simulink model "Taller5"  (R2024a)
settings: Solver=ode4  StartTime=0.0  StopTime=0.050  FixedStep=1e-6  RelTol=1e-3
values from neighbouring files (symbols this model uses):
  den = [1, R/L, 1/(L * Cap)]    [Taller5_codigo.m]
  Kd3 = 0.0362210629547162    (= 0.0362210629547)    [Taller5_codigo.m]
  Ki2 = 500    [Taller5_codigo.m]
  Ki3 = 1762.80242907617    (= 1762.80242908)    [Taller5_codigo.m]
  Kp = 100    [Taller5_codigo.m]
  Kp2 = 10    [Taller5_codigo.m]
  Kp3 = 16.7573383387027    (= 16.7573383387)    [Taller5_codigo.m]
  num = 1/(L * Cap)    (= 45454.5454545)    [Taller5_codigo.m]
libraries: slpidlib x2
settings Model: Creator=UsuarioF  LastModifiedBy=UsuarioF

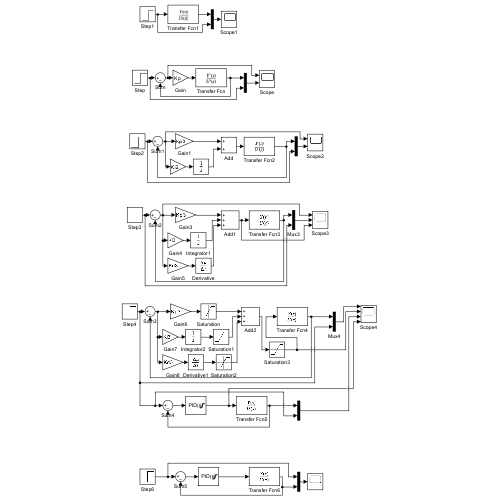
[thumbnail: Simulink's stored preview of the top-level diagram]
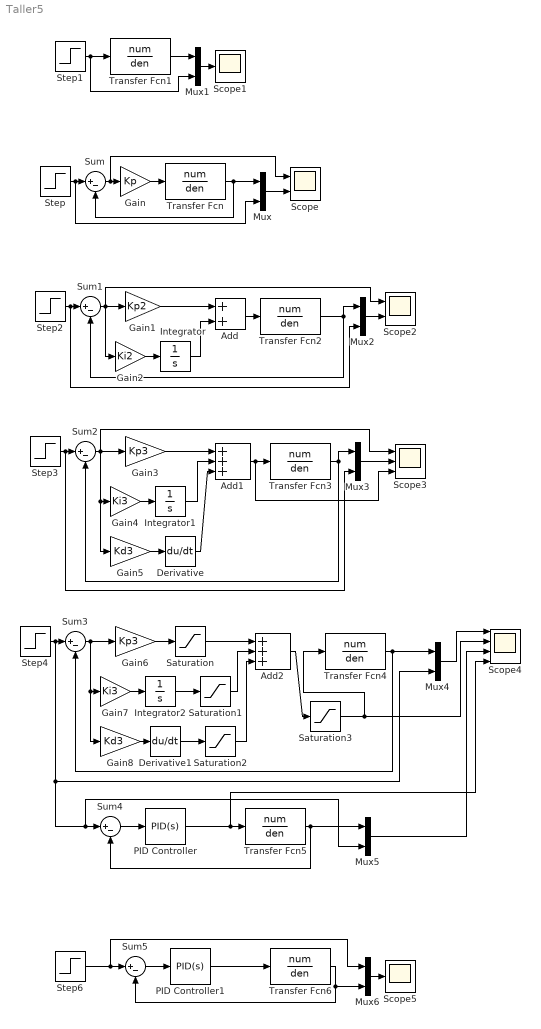
== system Taller5 ==
  Add : Sum
  Add1 : Sum  Inputs=+++
  Add2 : Sum  Inputs=+++
  Derivative : Derivative
  Derivative1 : Derivative
  Gain : Gain  Gain=Kp
  Gain1 : Gain  Gain=Kp2
  Gain2 : Gain  Gain=Ki2
  Gain3 : Gain  Gain=Kp3
  Gain4 : Gain  Gain=Ki3
  Gain5 : Gain  Gain=Kd3
  Gain6 : Gain  Gain=Kp3
  Gain7 : Gain  Gain=Ki3
  Gain8 : Gain  Gain=Kd3
  Integrator : Integrator
  Integrator1 : Integrator
  Integrator2 : Integrator
  Mux{,1..6} (7 alike) : Mux  Inputs=2
  PID Controller : slpidlib/PID Controller  Controller=PID  Form=Parallel  TimeDomain=Continuous-time  UseExternalTs=off  SampleTime=-1  IntegratorMethod=Forward Euler  FilterMethod=Forward Euler  ControllerParametersSource=internal  P=16.7573383387027  I=1762.80242907617  UseKiTs=off  D=0.0362210629547162  UseExternalDerivativeSource=off  N=6402.71206389871  UseFilter=on  TunerSelectOption=Transfer Function Based (PID Tuner App)  InitialConditionSource=internal  InitialConditionForIntegrator=0  InitialConditionForFilter=0  DifferentiatorICPrevScaledInput=0  ExternalReset=none  TrackingMode=off  Kt=1  LimitOutput=on  SatLimitsSource=internal  UpperSaturationLimit=15  LowerSaturationLimit=-15  LinearizeAsGain=on  AntiWindupMode=none  Kb=1  LimitIntegrator=off  UpperIntegratorSaturationLimit=inf  LowerIntegratorSaturationLimit=-inf  POutMin=[]  POutMax=[]  IOutMin=[]  IOutMax=[]  DOutMin=[]  DOutMax=[]  NOutMin=[]  NOutMax=[]  SumOutMin=[]  SumOutMax=[]  SaturationOutMin=[]  SaturationOutMax=[]  PParamMin=[]  PParamMax=[]  IParamMin=[]  IParamMax=[]  DParamMin=[]  DParamMax=[]  NParamMin=[]  NParamMax=[]  KbParamMin=[]  KbParamMax=[]  KtParamMin=[]  KtParamMax=[]  KbOutMin=[]  KbOutMax=[]  KtOutMin=[]  KtOutMax=[]  IntegratorOutMin=[]  IntegratorOutMax=[]  FilterOutMin=[]  FilterOutMax=[]  SumI1OutMin=[]  SumI1OutMax=[]  SumI2OutMin=[]  SumI2OutMax=[]  SumI3OutMin=[]  SumI3OutMax=[]  SumI4OutMin=[]  SumI4OutMax=[]  SumDOutMin=[]  SumDOutMax=[]  DifferentiatorOutMin=[]  DifferentiatorOutMax=[]  FilterDiffOutCoefMin=[]  FilterDiffOutCoefMax=[]  ReciprocalOutMin=[]  ReciprocalOutMax=[]  SumDenOutMin=[]  SumDenOutMax=[]  SumNumOutMin=[]  SumNumOutMax=[]  DivideOutMin=[]  DivideOutMax=[]  UdiffTsProdOutMin=[]  UdiffTsProdOutMax=[]  NTsProdOutMin=[]  NTsProdOutMax=[]  UintegralTsProdOutMin=[]  UintegralTsProdOutMax=[]  UngainTsProdOutMin=[]  UngainTsProdOutMax=[]  ClampingZeroOutDataTypeStr=Inherit: Inherit via back propagation  ClampingZeroOutMin=[]  ClampingZeroOutMax=[]  FilterDenConstantOutDataTypeStr=Inherit: Inherit via back propagation  FilterDenConstantOutMin=[]  FilterDenConstantOutMax=[]  PCopyOutDataTypeStr=Inherit: Inherit via back propagation  PCopyOutMin=[]  PCopyOutMax=[]  NCopyOutDataTypeStr=Inherit: Inherit via back propagation  NCopyOutMin=[]  NCopyOutMax=[]  IntegratorContinuousStateAttributes=''  IntegratorStateMustResolveToSignalObject=off  IntegratorRTWStateStorageClass=Auto  FilterContinuousStateAttributes=''  FilterStateMustResolveToSignalObject=off  FilterRTWStateStorageClass=Auto  ParallelPVariant=InternalParameters  IdealPVariant=Disabled  IVariant=InternalParameters  DVariant=InternalParameters  IntegratorVariant=Continuous  SatVariant=Enabled  AWVariant=Passthrough  PCopyVariant=Disabled  TRVariant=Disabled  FdbkBlocksVariant=Forward  IdealPFdbkVariant=Disabled  SatFdbkVariant=Disabled  DerivativeFilterVariant=ContFilter  NVariant=InternalParameters  NCopyVariant=Disabled  FilterICVariant=InternalICsFilter  IntegratorICVariant=InternalICs  ExternalResetVariant=Disabled  TRSumVariant=Passthrough  SumFdbkVariant=Disabled  SumVariant=Sum_PID  TsampFilterVariant=InternalTs  TsampNgainVariant=Passthrough  TsampIntegralVariant=Disabled_SignalSpec  ExternalSaturationOutDataTypeStr=Inherit: Same as second input  DerivativeSourceVariant=ErrorSignal
  PID Controller1 : slpidlib/PID Controller  Controller=PID  Form=Parallel  TimeDomain=Continuous-time  UseExternalTs=off  SampleTime=-1  IntegratorMethod=Forward Euler  FilterMethod=Forward Euler  ControllerParametersSource=internal  P=10  I=1000  UseKiTs=off  D=0.01  UseExternalDerivativeSource=off  N=1000000  UseFilter=on  TunerSelectOption=Transfer Function Based (PID Tuner App)  InitialConditionSource=internal  InitialConditionForIntegrator=0  InitialConditionForFilter=0  DifferentiatorICPrevScaledInput=0  ExternalReset=none  TrackingMode=off  Kt=1  LimitOutput=on  SatLimitsSource=internal  UpperSaturationLimit=15  LowerSaturationLimit=-15  LinearizeAsGain=on  AntiWindupMode=none  Kb=1  LimitIntegrator=off  UpperIntegratorSaturationLimit=inf  LowerIntegratorSaturationLimit=-inf  POutMin=[]  POutMax=[]  IOutMin=[]  IOutMax=[]  DOutMin=[]  DOutMax=[]  NOutMin=[]  NOutMax=[]  SumOutMin=[]  SumOutMax=[]  SaturationOutMin=[]  SaturationOutMax=[]  PParamMin=[]  PParamMax=[]  IParamMin=[]  IParamMax=[]  DParamMin=[]  DParamMax=[]  NParamMin=[]  NParamMax=[]  KbParamMin=[]  KbParamMax=[]  KtParamMin=[]  KtParamMax=[]  KbOutMin=[]  KbOutMax=[]  KtOutMin=[]  KtOutMax=[]  IntegratorOutMin=[]  IntegratorOutMax=[]  FilterOutMin=[]  FilterOutMax=[]  SumI1OutMin=[]  SumI1OutMax=[]  SumI2OutMin=[]  SumI2OutMax=[]  SumI3OutMin=[]  SumI3OutMax=[]  SumI4OutMin=[]  SumI4OutMax=[]  SumDOutMin=[]  SumDOutMax=[]  DifferentiatorOutMin=[]  DifferentiatorOutMax=[]  FilterDiffOutCoefMin=[]  FilterDiffOutCoefMax=[]  ReciprocalOutMin=[]  ReciprocalOutMax=[]  SumDenOutMin=[]  SumDenOutMax=[]  SumNumOutMin=[]  SumNumOutMax=[]  DivideOutMin=[]  DivideOutMax=[]  UdiffTsProdOutMin=[]  UdiffTsProdOutMax=[]  NTsProdOutMin=[]  NTsProdOutMax=[]  UintegralTsProdOutMin=[]  UintegralTsProdOutMax=[]  UngainTsProdOutMin=[]  UngainTsProdOutMax=[]  ClampingZeroOutDataTypeStr=Inherit: Inherit via back propagation  ClampingZeroOutMin=[]  ClampingZeroOutMax=[]  FilterDenConstantOutDataTypeStr=Inherit: Inherit via back propagation  FilterDenConstantOutMin=[]  FilterDenConstantOutMax=[]  PCopyOutDataTypeStr=Inherit: Inherit via back propagation  PCopyOutMin=[]  PCopyOutMax=[]  NCopyOutDataTypeStr=Inherit: Inherit via back propagation  NCopyOutMin=[]  NCopyOutMax=[]  IntegratorContinuousStateAttributes=''  IntegratorStateMustResolveToSignalObject=off  IntegratorRTWStateStorageClass=Auto  FilterContinuousStateAttributes=''  FilterStateMustResolveToSignalObject=off  FilterRTWStateStorageClass=Auto  ParallelPVariant=InternalParameters  IdealPVariant=Disabled  IVariant=InternalParameters  DVariant=InternalParameters  IntegratorVariant=Continuous  SatVariant=Enabled  AWVariant=Passthrough  PCopyVariant=Disabled  TRVariant=Disabled  FdbkBlocksVariant=Forward  IdealPFdbkVariant=Disabled  SatFdbkVariant=Disabled  DerivativeFilterVariant=ContFilter  NVariant=InternalParameters  NCopyVariant=Disabled  FilterICVariant=InternalICsFilter  IntegratorICVariant=InternalICs  ExternalResetVariant=Disabled  TRSumVariant=Passthrough  SumFdbkVariant=Disabled  SumVariant=Sum_PID  TsampFilterVariant=InternalTs  TsampNgainVariant=Passthrough  TsampIntegralVariant=Disabled_SignalSpec  ExternalSaturationOutDataTypeStr=Inherit: Same as second input  DerivativeSourceVariant=ErrorSignal
  Saturation{,1..3} (4 alike) : Saturate  UpperLimit=15  LowerLimit=-15
  Scope : Scope  NumInputPorts=2
  Scope1 : Scope
  Scope2 : Scope  NumInputPorts=2
  Scope3 : Scope  NumInputPorts=3
  Scope4 : Scope  NumInputPorts=4
  Scope5 : Scope
  Step{,1..4,6} (6 alike) : Step  Time=0.01  After=5  SampleTime=0  VectorParams1D=off
  Sum{,1..5} (6 alike) : Sum  Inputs=|+-
  Transfer Fcn{,1..6} (7 alike) : TransferFcn  Numerator=num  Denominator=den
  wires:
  Gain/1 -> Transfer Fcn/1
  Sum/1 -> Scope/1, Gain/1
  Step/1 -> Mux/2, Sum/1
  Transfer Fcn/1 -> Mux/1, Sum/2
  Mux/1 -> Scope/2
  Step1/1 -> Mux1/2, Transfer Fcn1/1
  Transfer Fcn1/1 -> Mux1/1
  Mux1/1 -> Scope1/1
  Mux2/1 -> Scope2/2
  Transfer Fcn2/1 -> Mux2/1, Sum1/2
  Sum1/1 -> Gain2/1, Scope2/1, Gain1/1
  Step2/1 -> Mux2/2, Sum1/1
  Gain2/1 -> Integrator/1
  Integrator/1 -> Add/2
  Gain1/1 -> Add/1
  Add/1 -> Transfer Fcn2/1
  Gain3/1 -> Add1/1
  Step3/1 -> Mux3/2, Sum2/1
  Sum2/1 -> Gain5/1, Gain4/1, Scope3/1, Gain3/1
  Mux3/1 -> Scope3/2
  Gain4/1 -> Integrator1/1
  Transfer Fcn3/1 -> Mux3/1, Sum2/2
  Integrator1/1 -> Add1/2
  Add1/1 -> Scope3/3, Transfer Fcn3/1
  Gain5/1 -> Derivative/1
  Derivative/1 -> Add1/3
  Gain8/1 -> Derivative1/1
  Transfer Fcn4/1 -> Mux4/1, Sum3/2
  Gain7/1 -> Integrator2/1
  Sum3/1 -> Gain8/1, Gain7/1, Gain6/1
  Gain6/1 -> Saturation/1
  Saturation/1 -> Add2/1
  Integrator2/1 -> Saturation1/1
  Derivative1/1 -> Saturation2/1
  Saturation1/1 -> Add2/2
  Saturation2/1 -> Add2/3
  Add2/1 -> Saturation3/1
  Saturation3/1 -> Scope4/2, Transfer Fcn4/1
  PID Controller/1 -> Scope4/4, Transfer Fcn5/1
  Sum4/1 -> PID Controller/1
  Transfer Fcn5/1 -> Sum4/2, Mux5/1
  Mux4/1 -> Scope4/1
  Mux5/1 -> Scope4/3
  Step4/1 -> Mux5/2, Sum4/1, Mux4/2, Sum3/1
  Step6/1 -> Mux6/1, Sum5/1
  Transfer Fcn6/1 -> Mux6/2, Sum5/2
  Sum5/1 -> PID Controller1/1
  PID Controller1/1 -> Transfer Fcn6/1
  Mux6/1 -> Scope5/1
